simulink model "p4_system_arch_master"  (R2020a)
settings: Solver=VariableStepAuto  StartTime=0.0  StopTime=10.0  RelTol=1e-3
(part 11 of 11)

== system p4_system_arch_master/System 10 : Electrical Distribution System /10.2 LV Distribution System /10.2.1	Internal LV Loom System/10.2.1.2	Inverter to Inverter LV connector loom system/Inverter Internal Wires/ETH_P Wire/10.2.1.2.20	Inverter internal wire "ETH_P" insulation ==

== system p4_system_arch_master/System 10 : Electrical Distribution System /10.2 LV Distribution System /10.2.1	Internal LV Loom System/10.2.1.2	Inverter to Inverter LV connector loom system/Inverter Internal Wires/GND Wire /10.2.1.2.09	Inverter internal wire "GND" ==

== system p4_system_arch_master/System 10 : Electrical Distribution System /10.2 LV Distribution System /10.2.1	Internal LV Loom System/10.2.1.2	Inverter to Inverter LV connector loom system/Inverter Internal Wires/GND Wire /10.2.1.2.21	Inverter internal wire "GND" insulation ==

== system p4_system_arch_master/System 10 : Electrical Distribution System /10.2 LV Distribution System /10.2.1	Internal LV Loom System/10.2.1.2	Inverter to Inverter LV connector loom system/Inverter Internal Wires/VCC Wire/10.2.1.2.03	Inverter internal wire "VCC" ==

== system p4_system_arch_master/System 10 : Electrical Distribution System /10.2 LV Distribution System /10.2.1	Internal LV Loom System/10.2.1.2	Inverter to Inverter LV connector loom system/Inverter Internal Wires/VCC Wire/10.2.1.2.15	Inverter internal wire "VCC" insulation ==

== system p4_system_arch_master/System 10 : Electrical Distribution System /10.2 LV Distribution System /10.2.1	Internal LV Loom System/10.2.1.1	Inverter to Motor LV loom system/Resolver sensor System/10.2.1.1.03	Resolver sensor  Wires/10.2.1.1.08	Resolver sensor  Wire Cos/10.2.1.1.07	Resolver sensor  Wire "Cos+" ==

== system p4_system_arch_master/System 10 : Electrical Distribution System /10.2 LV Distribution System /10.2.1	Internal LV Loom System/10.2.1.1	Inverter to Motor LV loom system/Resolver sensor System/10.2.1.1.03	Resolver sensor  Wires/10.2.1.1.08	Resolver sensor  Wire Cos/10.2.1.1.08	Resolver sensor  Wire "Cos-" ==

== system p4_system_arch_master/System 10 : Electrical Distribution System /10.2 LV Distribution System /10.2.1	Internal LV Loom System/10.2.1.1	Inverter to Motor LV loom system/Resolver sensor System/10.2.1.1.03	Resolver sensor  Wires/10.2.1.1.08	Resolver sensor  Wire Cos/10.2.1.1.13	Resolver sensor  Wire "Cos+" Insulation ==

== system p4_system_arch_master/System 10 : Electrical Distribution System /10.2 LV Distribution System /10.2.1	Internal LV Loom System/10.2.1.1	Inverter to Motor LV loom system/Resolver sensor System/10.2.1.1.03	Resolver sensor  Wires/10.2.1.1.08	Resolver sensor  Wire Cos/10.2.1.1.14	Resolver sensor  Wire "Cos-" Insulation ==

== system p4_system_arch_master/System 10 : Electrical Distribution System /10.2 LV Distribution System /10.2.1	Internal LV Loom System/10.2.1.1	Inverter to Motor LV loom system/Resolver sensor System/10.2.1.1.03	Resolver sensor  Wires/10.2.1.1.08	Resolver sensor  Wire Cos/10.2.1.1.17	Resolver sensor  Wire pair "Cos" shielding braid ==

== system p4_system_arch_master/System 10 : Electrical Distribution System /10.2 LV Distribution System /10.2.1	Internal LV Loom System/10.2.1.1	Inverter to Motor LV loom system/Resolver sensor System/10.2.1.1.03	Resolver sensor  Wires/Resolver sensor  Wire Sin/10.2.1.1.05	Resolver sensor  Wire "Sin-" ==

== system p4_system_arch_master/System 10 : Electrical Distribution System /10.2 LV Distribution System /10.2.1	Internal LV Loom System/10.2.1.1	Inverter to Motor LV loom system/Resolver sensor System/10.2.1.1.03	Resolver sensor  Wires/Resolver sensor  Wire Sin/10.2.1.1.06	Resolver sensor  Wire "Sin+" ==

== system p4_system_arch_master/System 10 : Electrical Distribution System /10.2 LV Distribution System /10.2.1	Internal LV Loom System/10.2.1.1	Inverter to Motor LV loom system/Resolver sensor System/10.2.1.1.03	Resolver sensor  Wires/Resolver sensor  Wire Sin/10.2.1.1.11	Resolver sensor  Wire "Sin-" Insulation ==

== system p4_system_arch_master/System 10 : Electrical Distribution System /10.2 LV Distribution System /10.2.1	Internal LV Loom System/10.2.1.1	Inverter to Motor LV loom system/Resolver sensor System/10.2.1.1.03	Resolver sensor  Wires/Resolver sensor  Wire Sin/10.2.1.1.12	Resolver sensor  Wire "Sin+" Insulation ==

== system p4_system_arch_master/System 10 : Electrical Distribution System /10.2 LV Distribution System /10.2.1	Internal LV Loom System/10.2.1.1	Inverter to Motor LV loom system/Resolver sensor System/10.2.1.1.03	Resolver sensor  Wires/Resolver sensor  Wire Sin/10.2.1.1.16	Resolver sensor  Wire pair "Sin" shielding braid ==

== system p4_system_arch_master/System 10 : Electrical Distribution System /10.2 LV Distribution System /10.2.1	Internal LV Loom System/10.2.1.1	Inverter to Motor LV loom system/Resolver sensor System/10.2.1.1.03	Resolver sensor  Wires/Resolver sensor Wire Ex/10.2.1.1.03	Resolver sensor  Wire "Ex+" ==

== system p4_system_arch_master/System 10 : Electrical Distribution System /10.2 LV Distribution System /10.2.1	Internal LV Loom System/10.2.1.1	Inverter to Motor LV loom system/Resolver sensor System/10.2.1.1.03	Resolver sensor  Wires/Resolver sensor Wire Ex/10.2.1.1.04	Resolver sensor  Wire "Ex-" ==

== system p4_system_arch_master/System 10 : Electrical Distribution System /10.2 LV Distribution System /10.2.1	Internal LV Loom System/10.2.1.1	Inverter to Motor LV loom system/Resolver sensor System/10.2.1.1.03	Resolver sensor  Wires/Resolver sensor Wire Ex/10.2.1.1.09	Resolver sensor  Wire "Ex+" Insulation ==

== system p4_system_arch_master/System 10 : Electrical Distribution System /10.2 LV Distribution System /10.2.1	Internal LV Loom System/10.2.1.1	Inverter to Motor LV loom system/Resolver sensor System/10.2.1.1.03	Resolver sensor  Wires/Resolver sensor Wire Ex/10.2.1.1.10	Resolver sensor  Wire "Ex-" Insulation ==

== system p4_system_arch_master/System 10 : Electrical Distribution System /10.2 LV Distribution System /10.2.1	Internal LV Loom System/10.2.1.1	Inverter to Motor LV loom system/Resolver sensor System/10.2.1.1.03	Resolver sensor  Wires/Resolver sensor Wire Ex/10.2.1.1.15	Resolver sensor  Wire pair "Ex" shielding braid ==
